simulink model "SecRwLtStLtwdRtwdCtrl"  (R2018b)
settings: Solver=FixedStepDiscrete  StartTime=0.0  StopTime=10.0  FixedStep=0.01  RelTol=1e-3
undefined symbols (not defined in the file or in its folder): KeSMSuMdMotFinshdTm_Val, KeSMSuMdRetryTm1_Val, KeSMSuModeReqDurgTm_Val, KeSMSwSecRwLtStLtwdRtwdEnTrigBitMask_Val
libraries: StCtrlLib x1
settings Model: Creator=sn2xws  LastModifiedBy=sn2xws
settings DataIOCC: SaveFormat=StructureWithTime
settings OptimizationCC: DefaultParameterBehavior=Inlined  EnhancedBackFolding=on  PassReuseOutputArgsAs=Individual arguments  ZeroExternalMemoryAtStartup=off  ZeroInternalMemoryAtStartup=off  OptimizeBlockOrder=speed  DifferentSizesBufferReuse=on  OptimizationCustomize=off
settings DebuggingCC: ParameterTunabilityLossMsg=error
settings ModelReferenceCC: ModelReferenceNumInstancesAllowed=Single
settings SFSimCC: MATLABDynamicMemAlloc=off
settings RTWCC: SystemTargetFile=autosar.tlc  GenCodeOnly=on  TemplateMakefile=ert_default_tmf  Description=AUTOSAR  GenerateReport=on  IncludeHyperlinkInReport=on  LaunchReport=on  GenerateTraceInfo=on  GenerateTraceReport=on  GenerateTraceReportSl=on  GenerateTraceReportSf=on  GenerateTraceReportEml=on
settings CodeAppCC: ForceParamTrailComments=on  IgnoreCustomStorageClasses=off  OperatorAnnotations=on  SimulinkDataObjDesc=on  SFDataObjDesc=on  InsertBlockDesc=on
settings STFCustomTargetCC: TargetLangStandard=C99 (ISO)  MultiwordLength=256  ParMdlRefBuildCompliant=on  CompOptLevelCompliant=on  IncludeMdlTerminateFcn=off  CombineOutputUpdateFcns=on  SuppressErrorStatus=on  ERTCustomFileBanners=on  SupportNonFinite=off  SupportComplex=off  SupportContinuousTime=off  SupportNonInlinedSFcns=off  RemoveResetFunc=on  MATLABClassNameForMDSCustomization=Simulink.SoftwareTarget.ERTCustomization  AutosarCompliant=on  UseToolchainInfoCompliant=on  LookupTableObjectStructAxisOrder=2,1,3,4,...  LUTObjectStructOrderEvenSpacing=Size,Table,Breakpoints  SystemTargetFile=autosar.tlc
settings ERTTargetCC: TargetLangStandard=C99 (ISO)  ConcurrentExecutionCompliant=off  IncludeMdlTerminateFcn=off  SuppressErrorStatus=on  SupportNonFinite=off  SupportComplex=off  ModelStepFunctionPrototypeControlCompliant=off  CPPClassGenCompliant=off  AutosarCompliant=on  LookupTableObjectStructAxisOrder=2,1,3,4,...  LUTObjectStructOrderEvenSpacing=Size,Table,Breakpoints  InlinedParameterPlacement=NonHierarchical  ERTCustomFileTemplate=example_file_process.tlc  ERTFilePackagingFormat=Compact

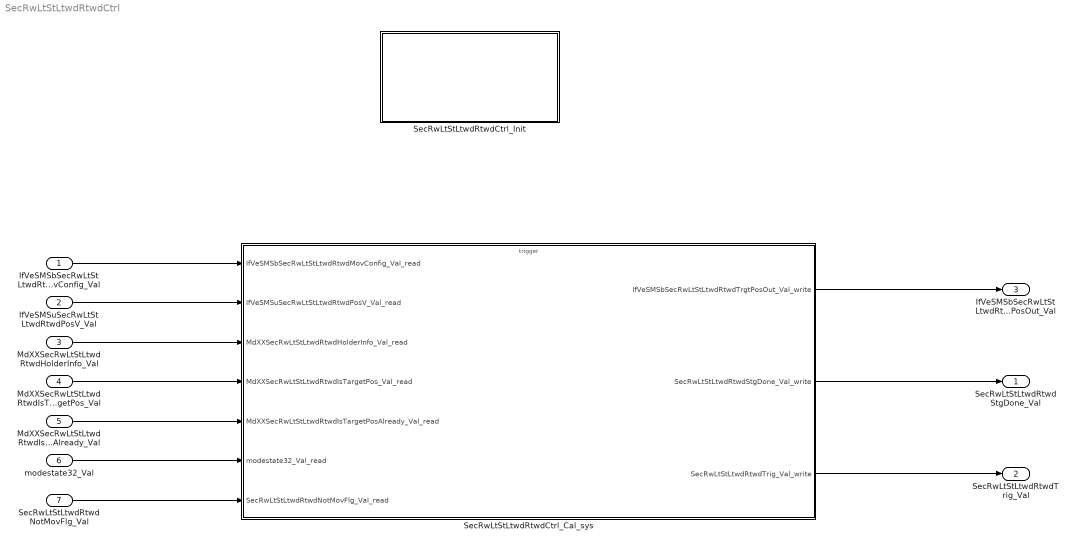
== system SecRwLtStLtwdRtwdCtrl ==
  IfVeSMSbSecRwLtStLtwdRtwdMovConfig_Val : Inport  OutDataTypeStr=boolean  PortDimensions=1
  IfVeSMSuSecRwLtStLtwdRtwdPosV_Val : Inport  Port=2  OutDataTypeStr=boolean  PortDimensions=1
  MdXXSecRwLtStLtwdRtwdHolderInfo_Val : Inport  Port=3  OutDataTypeStr=uint32  PortDimensions=1
  MdXXSecRwLtStLtwdRtwdIsTargetPos_Val : Inport  Port=4  OutDataTypeStr=uint32  PortDimensions=1
  MdXXSecRwLtStLtwdRtwdIsTargetPosAlready_Val : Inport  Port=5  OutDataTypeStr=uint32  PortDimensions=1
  modestate32_Val : Inport  Port=6  OutDataTypeStr=uint32  PortDimensions=1
  SecRwLtStLtwdRtwdNotMovFlg_Val : Inport  Port=7  OutDataTypeStr=boolean  PortDimensions=1
  SecRwLtStLtwdRtwdCtrl_Cal_sys : Subsystem
  SecRwLtStLtwdRtwdCtrl_Init : Subsystem
  SecRwLtStLtwdRtwdStgDone_Val : Outport  OutDataTypeStr=boolean  PortDimensions=1
  SecRwLtStLtwdRtwdTrig_Val : Outport  Port=2  OutDataTypeStr=boolean  PortDimensions=1
  IfVeSMSbSecRwLtStLtwdRtwdTrgtPosOut_Val : Outport  Port=3  OutDataTypeStr=boolean  PortDimensions=1
  wires:
  IfVeSMSbSecRwLtStLtwdRtwdMovConfig_Val/1 -> SecRwLtStLtwdRtwdCtrl_Cal_sys/1(IfVeSMSbSecRwLtStLtwdRtwdMovConfig_Val_read)
  IfVeSMSuSecRwLtStLtwdRtwdPosV_Val/1 -> SecRwLtStLtwdRtwdCtrl_Cal_sys/2(IfVeSMSuSecRwLtStLtwdRtwdPosV_Val_read)
  MdXXSecRwLtStLtwdRtwdHolderInfo_Val/1 -> SecRwLtStLtwdRtwdCtrl_Cal_sys/3(MdXXSecRwLtStLtwdRtwdHolderInfo_Val_read)
  MdXXSecRwLtStLtwdRtwdIsTargetPos_Val/1 -> SecRwLtStLtwdRtwdCtrl_Cal_sys/4(MdXXSecRwLtStLtwdRtwdIsTargetPos_Val_read)
  MdXXSecRwLtStLtwdRtwdIsTargetPosAlready_Val/1 -> SecRwLtStLtwdRtwdCtrl_Cal_sys/5(MdXXSecRwLtStLtwdRtwdIsTargetPosAlready_Val_read)
  modestate32_Val/1 -> SecRwLtStLtwdRtwdCtrl_Cal_sys/6(modestate32_Val_read)
  SecRwLtStLtwdRtwdNotMovFlg_Val/1 -> SecRwLtStLtwdRtwdCtrl_Cal_sys/7(SecRwLtStLtwdRtwdNotMovFlg_Val_read)
  SecRwLtStLtwdRtwdCtrl_Cal_sys/1(IfVeSMSbSecRwLtStLtwdRtwdTrgtPosOut_Val_write) -> IfVeSMSbSecRwLtStLtwdRtwdTrgtPosOut_Val/1
  SecRwLtStLtwdRtwdCtrl_Cal_sys/2(SecRwLtStLtwdRtwdStgDone_Val_write) -> SecRwLtStLtwdRtwdStgDone_Val/1
  SecRwLtStLtwdRtwdCtrl_Cal_sys/3(SecRwLtStLtwdRtwdTrig_Val_write) -> SecRwLtStLtwdRtwdTrig_Val/1

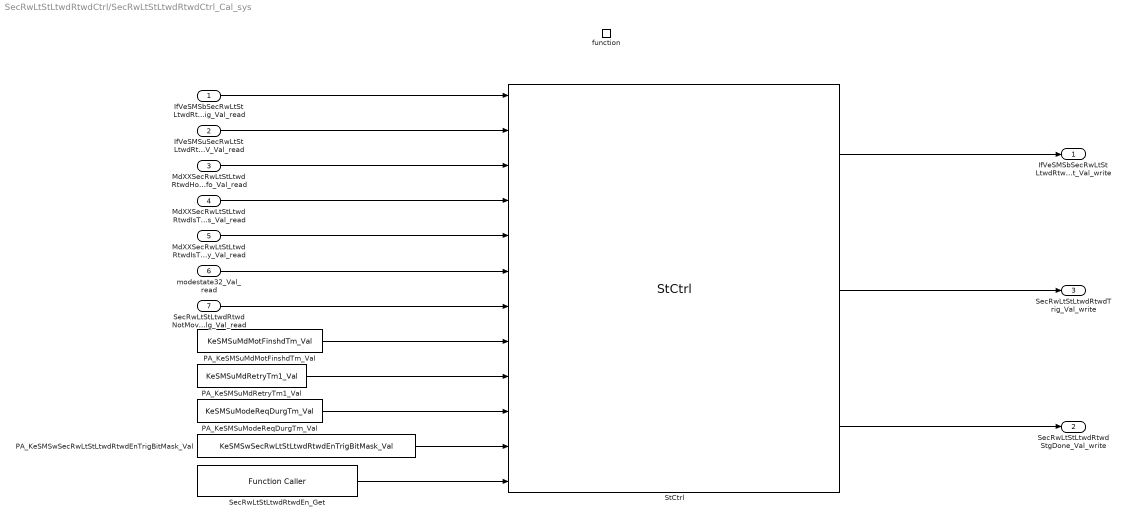
== system SecRwLtStLtwdRtwdCtrl/SecRwLtStLtwdRtwdCtrl_Cal_sys ==
  IfVeSMSbSecRwLtStLtwdRtwdMovConfig_Val_read : Inport
  IfVeSMSuSecRwLtStLtwdRtwdPosV_Val_read : Inport  Port=2
  MdXXSecRwLtStLtwdRtwdHolderInfo_Val_read : Inport  Port=3
  MdXXSecRwLtStLtwdRtwdIsTargetPos_Val_read : Inport  Port=4
  MdXXSecRwLtStLtwdRtwdIsTargetPosAlready_Val_read : Inport  Port=5
  modestate32_Val_read : Inport  Port=6
  SecRwLtStLtwdRtwdNotMovFlg_Val_read : Inport  Port=7
  function : TriggerPort  TriggerType=function-call  IsSimulinkFunction=on  FunctionName=SecRwLtStLtwdRtwdCtrl_Cal  VariantControl=(inherit)
  PA_KeSMSuMdMotFinshdTm_Val : Constant  Value=KeSMSuMdMotFinshdTm_Val
  PA_KeSMSuMdRetryTm1_Val : Constant  Value=KeSMSuMdRetryTm1_Val
  PA_KeSMSuModeReqDurgTm_Val : Constant  Value=KeSMSuModeReqDurgTm_Val
  PA_KeSMSwSecRwLtStLtwdRtwdEnTrigBitMask_Val : Constant  Value=KeSMSwSecRwLtStLtwdRtwdEnTrigBitMask_Val
  SecRwLtStLtwdRtwdEn_Get : FunctionCaller  FunctionPrototype=data = SecRwLtStLtwdRtwdEn_Get()  OutputArgumentSpecifications=uint32(1)
  StCtrl : StCtrlLib/StCtrl  SystemSampleTime=-1
  IfVeSMSbSecRwLtStLtwdRtwdTrgtPosOut_Val_write : Outport
      settings: EnsureOutportIsVirtual=on
  SecRwLtStLtwdRtwdStgDone_Val_write : Outport  Port=2
      settings: EnsureOutportIsVirtual=on
  SecRwLtStLtwdRtwdTrig_Val_write : Outport  Port=3
      settings: EnsureOutportIsVirtual=on
  wires:
  StCtrl/1 -> IfVeSMSbSecRwLtStLtwdRtwdTrgtPosOut_Val_write/1
  StCtrl/3 -> SecRwLtStLtwdRtwdStgDone_Val_write/1
  StCtrl/2 -> SecRwLtStLtwdRtwdTrig_Val_write/1
  PA_KeSMSwSecRwLtStLtwdRtwdEnTrigBitMask_Val/1 -> StCtrl/11
  SecRwLtStLtwdRtwdEn_Get/1 -> StCtrl/12
  PA_KeSMSuMdMotFinshdTm_Val/1 -> StCtrl/8
  PA_KeSMSuModeReqDurgTm_Val/1 -> StCtrl/10
  PA_KeSMSuMdRetryTm1_Val/1 -> StCtrl/9
  IfVeSMSbSecRwLtStLtwdRtwdMovConfig_Val_read/1 -> StCtrl/1
  IfVeSMSuSecRwLtStLtwdRtwdPosV_Val_read/1 -> StCtrl/2
  MdXXSecRwLtStLtwdRtwdHolderInfo_Val_read/1 -> StCtrl/3
  MdXXSecRwLtStLtwdRtwdIsTargetPos_Val_read/1 -> StCtrl/4
  MdXXSecRwLtStLtwdRtwdIsTargetPosAlready_Val_read/1 -> StCtrl/5
  modestate32_Val_read/1 -> StCtrl/6
  SecRwLtStLtwdRtwdNotMovFlg_Val_read/1 -> StCtrl/7

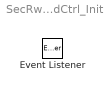
== system SecRwLtStLtwdRtwdCtrl/SecRwLtStLtwdRtwdCtrl_Init ==
  Event Listener : EventListener  EventName=reset
